simulink model "simulink_tri_motor_drone"  (R2020a)
settings: Solver=VariableStepAuto  StartTime=0.0  StopTime=50  RelTol=1e-3
values from neighbouring files (symbols this model uses):
  airDensity = 1.225    [tri_drone.m]
  areaWheelFront = wheelHeight*wheelWidth    (= 0.004)    [tri_drone.m]
  areaWing = 0.121    [tri_drone.m]
  cDFront = 0.9    [tri_drone.m]
  cDtable = [0.174 0.157 0.141 0.127 0.113 0.100 0.088 0.077 0.067 0.058 0.051 0.044 0.038 0.033 0.028 0.025 0.023 0.021 0.020 0.020 0.021 0.023 0.026 0.029 0.033 0.038 0.043 0.050 0.056 0.064 0.072 0.081 0.091 0.101 0.112 0.124 0.137 0.150 0.165 0.180 0.196 0.212 0.229 0.245 0.261 0.277 0.292 0.306 0.319 0.331 0.341]    [tri_drone.m]
  cLtable = [-1.07 -1.02 -0.97 -0.92 -0.87 -0.81 -0.76 -0.70 -0.65 -0.59 -0.54 -0.48 -0.43 -0.37 -0.31 -0.25 -0.19 -0.13 -0.07 -0.01 0.05 0.11 0.17 0.23 0.29 0.35 0.40 0.46 0.52 0.57 0.63 0.68 0.74 0.79 0.85 0.90 0.95 1.00 1.05 1.10 1.15 1.20 1.25 1.29 1.32 1.36 1.38 1.41 1.43 1.44 1.45]    [tri_drone.m]
  heightRef = 1.0    (= 1)    [tri_drone.m]
  hoverRot = w(11)    [tri_drone.m]
  hoverVel = trustPerPropeller / Ktrust /pi * 180.0    [tri_drone.m]
  hoverVoltagefine = 0.35*11.9    (= 4.165)    [tri_drone.m]
  KDheightcoarse = 15.0    (= 15)    [tri_drone.m]
  KDheightfine = 0    [tri_drone.m]
  KDrag = 8 * (ampMax * Km / (rpmMax / 60 * 2 * pi))    (= 0.000150440801971)    [tri_drone.m]
  KIheightcoarse = 5.0    (= 5)    [tri_drone.m]
  KIheightfine = 0    [tri_drone.m]
  Km = 60/(Kv * 2 * pi)    (= 0.00415186808066)    [tri_drone.m]
  KPheightcoarse = 0.1    [tri_drone.m]
  KPheightfine = 0    [tri_drone.m]
  Ktrust = (trustMax * g)/(rpmMax / 60 * 2 * pi)    (= 0.00223215912077)    [tri_drone.m]
  mBodyTotal = 0.422 + mBattery    (= 0.797)    [tri_drone.m]
  motorMass = 0.022    [tri_drone.m]
  N = 1000000    [tri_drone.m]
  pitch_lower_limit = theta(1)    [tri_drone.m]
  pitch_upper_limit = theta(end)    [tri_drone.m]
  propellerMass = 0.012    [tri_drone.m]
  Ra = RaVolt/ampMax    (= 0.133333333333)    [tri_drone.m]
  rInner = armRadius    (= 0.27)    [tri_drone.m]
  rOuter = armRadius + wLength    (= 0.91)    [tri_drone.m]
  theta = [-10 -9.5 -9.0 -8.5 -8.0 -7.5 -7.0 -6.5 -6.0 -5.5 -5.0 -4.5 -4.0 -3.5 -3.0 -2.5 -2.0 -1.5 -1.0 -0.5 0 0.5 1.0 1.5 2.0 2.5 3.0 3.5 4.0 4.5 5.0 5.5 6.0 6.5 7.0 7.5 8.0 8.5 9.0 9.5 10.0 10.5 11.0 11.5 12.0 12.5 13.0 13.5 14.0 14.5 15.0]    [tri_drone.m]
  Ts = 0.002    [tri_drone.m]
  Ts2 = 0.03    [tri_drone.m]
  wHeight = 0.025    [tri_drone.m]
  wingDensity = 50    [tri_drone.m]
  wLength = 0.64    [tri_drone.m]
  wWidth = 0.20    (= 0.2)    [tri_drone.m]
undefined symbols (not defined in the file or in its folder): X, Y, Z
libraries: sm_lib x53, nesl_utility x45
(part 3 of 3)

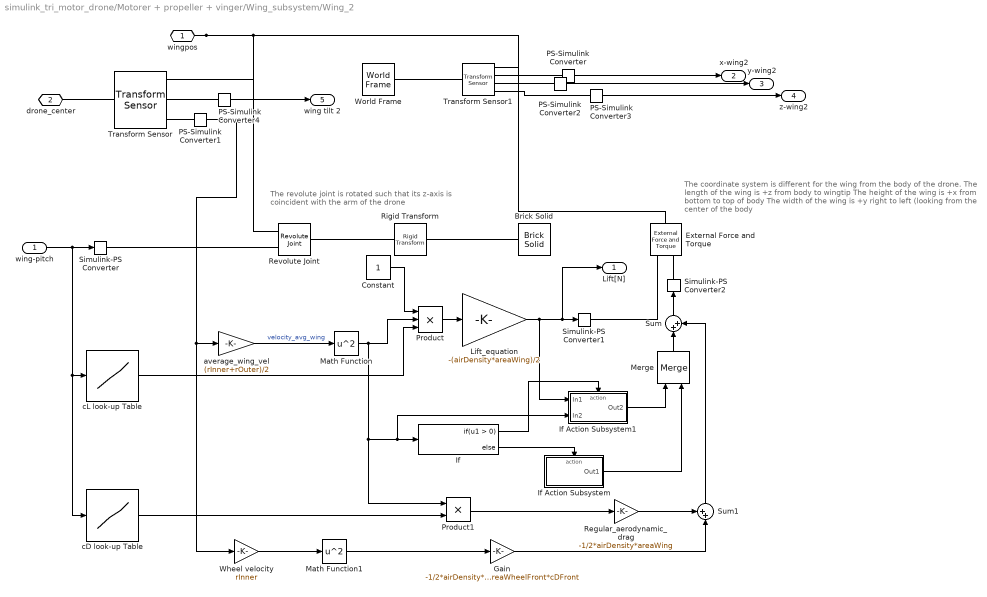
== system simulink_tri_motor_drone/Motorer + propeller + vinger/Wing_subsystem/Wing_2 ==
  note: The revolute joint is rotated such that its z-axis is
      | coincident with the arm of the drone
  note: The coordinate system is different for the wing from the body of the drone.
      | The length of the wing is +z from body to wingtip
      | The height of the wing is +x from bottom to top of body
      | The width of the wing is +y right to left (looking from the center of the body
  wing-pitch : Inport
  Brick Solid : sm_lib/Body Elements/Brick Solid  GraphicAmbientColor=[0.15 0.15 0.15 1.0]  BasedOnType=Mass  BrickDimensions=[wWidth wLength wHeight]  BrickDimensionUnits=m  CenterOfMass=[0 0 0]  CenterOfMassUnits=m  GraphicDiffuseColor=[1.0 0.0 0.2]  Density=wingDensity  DensityUnits=kg/m^3  DoExposeReferenceFrame=on  GraphicEmissiveColor=[0.0 0.0 0.0 1.0]  ExportEntireGeometry=off  SerializedFrames=<Frames/>  MarkerShape=Sphere  MarkerSize=10  GraphicType=FromGeometry  InertiaType=CalculateFromGeometry  Mass=areaWing*wHeight*wingDensity  MassUnits=kg  MomentsOfInertia=[1 1 1]  MomentsOfInertiaUnits=kg*m^2  GraphicOpacity=1.0  ProductsOfInertia=[0 0 0]  ProductsOfInertiaUnits=kg*m^2  GraphicShininess=75  GraphicSpecularColor=[0.5 0.5 0.5 1.0]  GraphicVisPropType=SimpleVisualProperties
  Constant : Constant
  External Force and Torque : sm_lib/Forces and Torques/External Force and Torque  ForceResolutionFrame=AttachedFrame  EnableForceX=on  EnableForceY=on  EnableForceZ=off  EnableForce=off  TorqueResolutionFrame=AttachedFrame  EnableTorqueX=off  EnableTorqueY=off  EnableTorqueZ=off  EnableTorque=off
  Gain : Gain  Gain=-1/2*airDensity*areaWheelFront*cDFront
  If : If
  If Action Subsystem : Subsystem  TreatAsAtomicUnit=on
  If Action Subsystem1 : Subsystem  TreatAsAtomicUnit=on
  Lift_equation : Gain  Gain=-(airDensity*areaWing)/2
  Math Function : Math  Operator=square  SaturateOnIntegerOverflow=on
  Math Function1 : Math  Operator=square  SaturateOnIntegerOverflow=on
  Merge : Merge
  PS-Simulink Converter{,1..4} (5 alike) : nesl_utility/PS-Simulink Converter  PhysicalDomain=network_engine_domain  SubClassName=ps_output  LeftPortType=input  RightPortType=output  PseudoPeriodic=off  Frequencies=[]  Unit=inherit  AffineConversion=off
  Product : Product  Inputs=3
  Product1 : Product
  Regular_aerodynamic_drag : Gain  Gain=-1/2*airDensity*areaWing
  Revolute Joint : sm_lib/Joints/Revolute Joint  JointMode=Normal  SenseConstraintForce=off  SenseConstraintForceX=off  SenseConstraintForceY=off  SenseConstraintForceZ=off  SenseConstraintTorque=off  SenseConstraintTorqueX=off  SenseConstraintTorqueY=off  SenseConstraintTorqueZ=off  SenseTotalForce=off  SenseTotalForceX=off  SenseTotalForceY=off  SenseTotalForceZ=off  SenseTotalTorque=off  SenseTotalTorqueX=off  SenseTotalTorqueY=off  SenseTotalTorqueZ=off  CompositeWrenchDir=FollowerOnBase  CompositeWrenchFrame=BaseFrame  EquilibriumPosition=0  EquilibriumPositionUnits=deg  SpringStiffness=0  SpringStiffnessUnits=N*m/deg  DampingCoefficient=0  DampingCoefficientUnits=N*m/(deg/s)  TorqueActuationMode=ComputedTorque  MotionActuationMode=InputMotion  SensePosition=off  SenseVelocity=off  SenseAcceleration=off  SenseTorqueForce=off  SenseLowerLimitTorqueForce=off  SenseUpperLimitTorqueForce=off  LowerLimitSpecify=off  LowerLimitBound=-90  LowerLimitBoundUnits=deg  LowerLimitStiffness=1e4  LowerLimitStiffnessUnits=N*m/deg  LowerLimitDamping=10  LowerLimitDampingUnits=N*m/(deg/s)  LowerLimitTransitionRegionWidth=0.1  LowerLimitTransitionRegionWidthUnits=deg  UpperLimitSpecify=off  UpperLimitBound=90  UpperLimitBoundUnits=deg  UpperLimitStiffness=1e4  UpperLimitStiffnessUnits=N*m/deg  UpperLimitDamping=10  UpperLimitDampingUnits=N*m/(deg/s)  UpperLimitTransitionRegionWidth=0.1  UpperLimitTransitionRegionWidthUnits=deg  PositionTargetSpecify=off  PositionTargetPriority=High  PositionTargetValue=0  PositionTargetValueUnits=deg  VelocityTargetSpecify=off  VelocityTargetPriority=High  VelocityTargetValue=0  VelocityTargetValueUnits=deg/s
  Rigid Transform : sm_lib/Frames and Transforms/Rigid Transform  TranslationMethod=Cartesian  TranslationStandardOffset=0  TranslationLengthUnit=m  TranslationStandardAxis=+Z  TranslationCartesianOffset=[0 0 wLength/2]  TranslationROffset=0  TranslationROffsetUnits=m  TranslationZOffset=0  TranslationZOffsetUnits=m  TranslationThetaOffset=0  TranslationThetaOffsetUnits=deg  RotationMethod=RotationSequence  RotationAngleUnits=deg  RotationStandardAxis=+Z  RotationAngle=0.0  RotationArbitraryAxis=[0 0 1]  FollAlignAxisA=+X  BaseAlignAxisA=+Y  FollAlignAxisB=+Y  BaseAlignAxisB=+Z  RotationSequenceAxes=FollowerAxes  RotationSequence=XZY  RotationSequenceAngles=[90 0 90]  RotationSequenceAnglesUnits=deg  RotationMatrix=[1 0 0; 0 1 0; 0 0 1]
  Simulink-PS Converter : nesl_utility/Simulink-PS Converter  PhysicalDomain=network_engine_domain  SubClassName=ps_input  LeftPortType=input  RightPortType=output  PseudoPeriodic=off  Frequencies=[]  NoiseDistribution=none  NoiseParameters=[]  Unit=deg  AffineConversion=off  FilteringAndDerivatives=filter  SimscapeFilterOrder=2  InputFilterTimeConstant=0.001  UdotUserProvided=0
  Simulink-PS Converter1 : nesl_utility/Simulink-PS Converter  PhysicalDomain=network_engine_domain  SubClassName=ps_input  LeftPortType=input  RightPortType=output  PseudoPeriodic=off  Frequencies=[]  NoiseDistribution=none  NoiseParameters=[]  Unit=1  AffineConversion=off  FilteringAndDerivatives=provide  SimscapeFilterOrder=1  InputFilterTimeConstant=0.001  UdotUserProvided=0
  Simulink-PS Converter2 : nesl_utility/Simulink-PS Converter  PhysicalDomain=network_engine_domain  SubClassName=ps_input  LeftPortType=input  RightPortType=output  PseudoPeriodic=off  Frequencies=[]  NoiseDistribution=none  NoiseParameters=[]  Unit=1  AffineConversion=off  FilteringAndDerivatives=provide  SimscapeFilterOrder=1  InputFilterTimeConstant=0.001  UdotUserProvided=0
  Sum : Sum  Inputs=|++
  Sum1 : Sum  Inputs=++|
  Transform Sensor : sm_lib/Frames and Transforms/Transform Sensor  MeasurementFrame=World  SenseAngle=on  SenseAxis=off  SenseAngle1=off  SenseAngle2=off  SenseAngle3=off  SenseQ=off  SenseR=off  SenseOmegaX=off  SenseOmegaY=off  SenseOmegaZ=on  SenseOmega1=off  SenseOmega2=off  SenseOmega3=off  SenseQDot=off  SenseRDot=off  SenseAlphaX=off  SenseAlphaY=off  SenseAlphaZ=off  SenseAlpha1=off  SenseAlpha2=off  SenseAlpha3=off  SenseQDDot=off  SenseRDDot=off  SenseX=off  SenseY=off  SenseZ=off  SenseRad=off  SenseAzim=off  SenseDist=off  SenseInc=off  SenseXDot=off  SenseYDot=off  SenseZDot=off  SenseRadDot=off  SenseAzimDot=off  SenseDistDot=off  SenseIncDot=off  SenseXDDot=off  SenseYDDot=off  SenseZDDot=off  SenseRadDDot=off  SenseAzimDDot=off  SenseDistDDot=off  SenseIncDDot=off
  Transform Sensor1 : sm_lib/Frames and Transforms/Transform Sensor  MeasurementFrame=World  SenseAngle=off  SenseAxis=off  SenseAngle1=off  SenseAngle2=off  SenseAngle3=off  SenseQ=off  SenseR=off  SenseOmegaX=off  SenseOmegaY=off  SenseOmegaZ=off  SenseOmega1=off  SenseOmega2=off  SenseOmega3=off  SenseQDot=off  SenseRDot=off  SenseAlphaX=off  SenseAlphaY=off  SenseAlphaZ=off  SenseAlpha1=off  SenseAlpha2=off  SenseAlpha3=off  SenseQDDot=off  SenseRDDot=off  SenseX=on  SenseY=on  SenseZ=on  SenseRad=off  SenseAzim=off  SenseDist=off  SenseInc=off  SenseXDot=off  SenseYDot=off  SenseZDot=off  SenseRadDot=off  SenseAzimDot=off  SenseDistDot=off  SenseIncDot=off  SenseXDDot=off  SenseYDDot=off  SenseZDDot=off  SenseRadDDot=off  SenseAzimDDot=off  SenseDistDDot=off  SenseIncDDot=off
  Wheel velocity : Gain  Gain=rInner
  World Frame : sm_lib/Frames and Transforms/World Frame
  average_wing_vel : Gain  Gain=(rInner+rOuter)/2
  cD look-up Table : Lookup_n-D  NumberOfTableDimensions=1  BreakpointsForDimension1=theta  Table=cDtable  InternalRulePriority=Speed  RndMeth=Simplest  InputSameDT=on
  cL look-up Table : Lookup_n-D  NumberOfTableDimensions=1  BreakpointsForDimension1=theta  Table=cLtable  InternalRulePriority=Speed  RndMeth=Simplest  InputSameDT=on
  wingpos : PMIOPort  Side=Left
  drone_center : PMIOPort  Port=2  Side=Left
  Lift[N] : Outport
  x-wing2 : Outport  Port=2
  y-wing2 : Outport  Port=3
  z-wing2 : Outport  Port=4
  wing tilt 2 : Outport  Port=5
  wires:
  wing-pitch/1 -> cD look-up Table/1, cL look-up Table/1, Simulink-PS Converter/1
  average_wing_vel/1 -> Math Function/1  "velocity_avg_wing"
  Product/1 -> Lift_equation/1
  PS-Simulink Converter/1 -> x-wing2/1
  PS-Simulink Converter2/1 -> y-wing2/1
  PS-Simulink Converter3/1 -> z-wing2/1
  cL look-up Table/1 -> Product/3
  Math Function/1 -> Product1/1, If Action Subsystem1/2(In2), If/1, Product/2
  If/1 -> If Action Subsystem1/Action
  If/2 -> If Action Subsystem/Action
  If Action Subsystem/1(Out1) -> Merge/2
  If Action Subsystem1/1(Out2) -> Merge/1
  Lift_equation/1 -> If Action Subsystem1/1(In1), Lift[N]/1, Simulink-PS Converter1/1
  Sum/1 -> Simulink-PS Converter2/1
  Merge/1 -> Sum/1
  PS-Simulink Converter4/1 -> wing tilt 2/1
  cD look-up Table/1 -> Product1/2
  Product1/1 -> Regular_aerodynamic_drag/1
  Constant/1 -> Product/1
  Gain/1 -> Sum1/2
  Wheel velocity/1 -> Math Function1/1
  PS-Simulink Converter1/1 -> Wheel velocity/1, average_wing_vel/1
  Math Function1/1 -> Gain/1
  Regular_aerodynamic_drag/1 -> Sum1/1
  Sum1/1 -> Sum/2
  connections:
  wingpos/RConn1 -- External Force and Torque/RConn1 -- Transform Sensor1/RConn1 -- Revolute Joint/LConn1 -- Transform Sensor/RConn1
  Revolute Joint/LConn2 -- Simulink-PS Converter/RConn1
  Rigid Transform/RConn1 -- Brick Solid/RConn1
  drone_center/RConn1 -- Transform Sensor/LConn1
  External Force and Torque/LConn1 -- Simulink-PS Converter1/RConn1
  World Frame/RConn1 -- Transform Sensor1/LConn1
  PS-Simulink Converter/LConn1 -- Transform Sensor1/RConn2
  Transform Sensor1/RConn3 -- PS-Simulink Converter2/LConn1
  Transform Sensor1/RConn4 -- PS-Simulink Converter3/LConn1
  Rigid Transform/LConn1 -- Revolute Joint/RConn1
  Simulink-PS Converter2/RConn1 -- External Force and Torque/LConn2
  Transform Sensor/RConn3 -- PS-Simulink Converter1/LConn1
  Transform Sensor/RConn2 -- PS-Simulink Converter4/LConn1

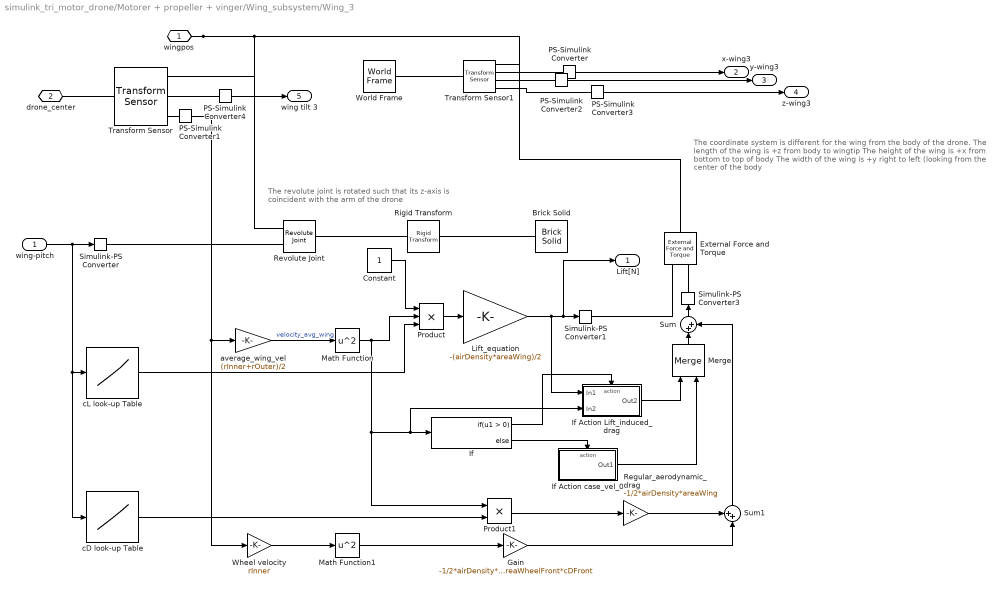
== system simulink_tri_motor_drone/Motorer + propeller + vinger/Wing_subsystem/Wing_3 ==
  note: The revolute joint is rotated such that its z-axis is
      | coincident with the arm of the drone
  note: The coordinate system is different for the wing from the body of the drone.
      | The length of the wing is +z from body to wingtip
      | The height of the wing is +x from bottom to top of body
      | The width of the wing is +y right to left (looking from the center of the body
  wing-pitch : Inport
  Brick Solid : sm_lib/Body Elements/Brick Solid  GraphicAmbientColor=[0.15 0.15 0.15 1.0]  BasedOnType=Mass  BrickDimensions=[wWidth wLength wHeight]  BrickDimensionUnits=m  CenterOfMass=[0 0 0]  CenterOfMassUnits=m  GraphicDiffuseColor=[1.0 0.8 0.0]  Density=wingDensity  DensityUnits=kg/m^3  DoExposeReferenceFrame=on  GraphicEmissiveColor=[0.0 0.0 0.0 1.0]  ExportEntireGeometry=off  SerializedFrames=<Frames/>  MarkerShape=Sphere  MarkerSize=10  GraphicType=FromGeometry  InertiaType=CalculateFromGeometry  Mass=areaWing*wHeight*wingDensity  MassUnits=kg  MomentsOfInertia=[1 1 1]  MomentsOfInertiaUnits=kg*m^2  GraphicOpacity=1.0  ProductsOfInertia=[0 0 0]  ProductsOfInertiaUnits=kg*m^2  GraphicShininess=75  GraphicSpecularColor=[0.5 0.5 0.5 1.0]  GraphicVisPropType=SimpleVisualProperties
  Constant : Constant
  External Force and Torque : sm_lib/Forces and Torques/External Force and Torque  ForceResolutionFrame=AttachedFrame  EnableForceX=on  EnableForceY=on  EnableForceZ=off  EnableForce=off  TorqueResolutionFrame=AttachedFrame  EnableTorqueX=off  EnableTorqueY=off  EnableTorqueZ=off  EnableTorque=off
  Gain : Gain  Gain=-1/2*airDensity*areaWheelFront*cDFront
  If : If
  If Action Lift_induced_drag : Subsystem  TreatAsAtomicUnit=on
  If Action case_vel_0 : Subsystem  TreatAsAtomicUnit=on
  Lift_equation : Gain  Gain=-(airDensity*areaWing)/2
  Math Function : Math  Operator=square  SaturateOnIntegerOverflow=on
  Math Function1 : Math  Operator=square  SaturateOnIntegerOverflow=on
  Merge : Merge  InitialOutput=0
  PS-Simulink Converter{,1..4} (5 alike) : nesl_utility/PS-Simulink Converter  PhysicalDomain=network_engine_domain  SubClassName=ps_output  LeftPortType=input  RightPortType=output  PseudoPeriodic=off  Frequencies=[]  Unit=inherit  AffineConversion=off
  Product : Product  Inputs=3
  Product1 : Product
  Regular_aerodynamic_drag : Gain  Gain=-1/2*airDensity*areaWing
  Revolute Joint : sm_lib/Joints/Revolute Joint  JointMode=Normal  SenseConstraintForce=off  SenseConstraintForceX=off  SenseConstraintForceY=off  SenseConstraintForceZ=off  SenseConstraintTorque=off  SenseConstraintTorqueX=off  SenseConstraintTorqueY=off  SenseConstraintTorqueZ=off  SenseTotalForce=off  SenseTotalForceX=off  SenseTotalForceY=off  SenseTotalForceZ=off  SenseTotalTorque=off  SenseTotalTorqueX=off  SenseTotalTorqueY=off  SenseTotalTorqueZ=off  CompositeWrenchDir=FollowerOnBase  CompositeWrenchFrame=BaseFrame  EquilibriumPosition=0  EquilibriumPositionUnits=deg  SpringStiffness=0  SpringStiffnessUnits=N*m/deg  DampingCoefficient=0  DampingCoefficientUnits=N*m/(deg/s)  TorqueActuationMode=ComputedTorque  MotionActuationMode=InputMotion  SensePosition=off  SenseVelocity=off  SenseAcceleration=off  SenseTorqueForce=off  SenseLowerLimitTorqueForce=off  SenseUpperLimitTorqueForce=off  LowerLimitSpecify=off  LowerLimitBound=-90  LowerLimitBoundUnits=deg  LowerLimitStiffness=1e4  LowerLimitStiffnessUnits=N*m/deg  LowerLimitDamping=10  LowerLimitDampingUnits=N*m/(deg/s)  LowerLimitTransitionRegionWidth=0.1  LowerLimitTransitionRegionWidthUnits=deg  UpperLimitSpecify=off  UpperLimitBound=90  UpperLimitBoundUnits=deg  UpperLimitStiffness=1e4  UpperLimitStiffnessUnits=N*m/deg  UpperLimitDamping=10  UpperLimitDampingUnits=N*m/(deg/s)  UpperLimitTransitionRegionWidth=0.1  UpperLimitTransitionRegionWidthUnits=deg  PositionTargetSpecify=off  PositionTargetPriority=High  PositionTargetValue=0  PositionTargetValueUnits=deg  VelocityTargetSpecify=off  VelocityTargetPriority=High  VelocityTargetValue=0  VelocityTargetValueUnits=deg/s
  Rigid Transform : sm_lib/Frames and Transforms/Rigid Transform  TranslationMethod=Cartesian  TranslationStandardOffset=0  TranslationLengthUnit=m  TranslationStandardAxis=+Z  TranslationCartesianOffset=[0 0 wLength/2]  TranslationROffset=0  TranslationROffsetUnits=m  TranslationZOffset=0  TranslationZOffsetUnits=m  TranslationThetaOffset=0  TranslationThetaOffsetUnits=deg  RotationMethod=RotationSequence  RotationAngleUnits=deg  RotationStandardAxis=+Z  RotationAngle=0.0  RotationArbitraryAxis=[0 0 1]  FollAlignAxisA=+X  BaseAlignAxisA=+Y  FollAlignAxisB=+Y  BaseAlignAxisB=+Z  RotationSequenceAxes=FollowerAxes  RotationSequence=XZY  RotationSequenceAngles=[90 0 90]  RotationSequenceAnglesUnits=deg  RotationMatrix=[1 0 0; 0 1 0; 0 0 1]
  Simulink-PS Converter : nesl_utility/Simulink-PS Converter  PhysicalDomain=network_engine_domain  SubClassName=ps_input  LeftPortType=input  RightPortType=output  PseudoPeriodic=off  Frequencies=[]  NoiseDistribution=none  NoiseParameters=[]  Unit=deg  AffineConversion=off  FilteringAndDerivatives=filter  SimscapeFilterOrder=2  InputFilterTimeConstant=0.001  UdotUserProvided=0
  Simulink-PS Converter1 : nesl_utility/Simulink-PS Converter  PhysicalDomain=network_engine_domain  SubClassName=ps_input  LeftPortType=input  RightPortType=output  PseudoPeriodic=off  Frequencies=[]  NoiseDistribution=none  NoiseParameters=[]  Unit=1  AffineConversion=off  FilteringAndDerivatives=provide  SimscapeFilterOrder=1  InputFilterTimeConstant=0.001  UdotUserProvided=0
  Simulink-PS Converter3 : nesl_utility/Simulink-PS Converter  PhysicalDomain=network_engine_domain  SubClassName=ps_input  LeftPortType=input  RightPortType=output  PseudoPeriodic=off  Frequencies=[]  NoiseDistribution=none  NoiseParameters=[]  Unit=1  AffineConversion=off  FilteringAndDerivatives=provide  SimscapeFilterOrder=1  InputFilterTimeConstant=0.001  UdotUserProvided=0
  Sum : Sum  Inputs=|++
  Sum1 : Sum  Inputs=++|
  Transform Sensor : sm_lib/Frames and Transforms/Transform Sensor  MeasurementFrame=Base  SenseAngle=on  SenseAxis=off  SenseAngle1=off  SenseAngle2=off  SenseAngle3=off  SenseQ=off  SenseR=off  SenseOmegaX=off  SenseOmegaY=off  SenseOmegaZ=on  SenseOmega1=off  SenseOmega2=off  SenseOmega3=off  SenseQDot=off  SenseRDot=off  SenseAlphaX=off  SenseAlphaY=off  SenseAlphaZ=off  SenseAlpha1=off  SenseAlpha2=off  SenseAlpha3=off  SenseQDDot=off  SenseRDDot=off  SenseX=off  SenseY=off  SenseZ=off  SenseRad=off  SenseAzim=off  SenseDist=off  SenseInc=off  SenseXDot=off  SenseYDot=off  SenseZDot=off  SenseRadDot=off  SenseAzimDot=off  SenseDistDot=off  SenseIncDot=off  SenseXDDot=off  SenseYDDot=off  SenseZDDot=off  SenseRadDDot=off  SenseAzimDDot=off  SenseDistDDot=off  SenseIncDDot=off
  Transform Sensor1 : sm_lib/Frames and Transforms/Transform Sensor  MeasurementFrame=World  SenseAngle=off  SenseAxis=off  SenseAngle1=off  SenseAngle2=off  SenseAngle3=off  SenseQ=off  SenseR=off  SenseOmegaX=off  SenseOmegaY=off  SenseOmegaZ=off  SenseOmega1=off  SenseOmega2=off  SenseOmega3=off  SenseQDot=off  SenseRDot=off  SenseAlphaX=off  SenseAlphaY=off  SenseAlphaZ=off  SenseAlpha1=off  SenseAlpha2=off  SenseAlpha3=off  SenseQDDot=off  SenseRDDot=off  SenseX=on  SenseY=on  SenseZ=on  SenseRad=off  SenseAzim=off  SenseDist=off  SenseInc=off  SenseXDot=off  SenseYDot=off  SenseZDot=off  SenseRadDot=off  SenseAzimDot=off  SenseDistDot=off  SenseIncDot=off  SenseXDDot=off  SenseYDDot=off  SenseZDDot=off  SenseRadDDot=off  SenseAzimDDot=off  SenseDistDDot=off  SenseIncDDot=off
  Wheel velocity : Gain  Gain=rInner
  World Frame : sm_lib/Frames and Transforms/World Frame
  average_wing_vel : Gain  Gain=(rInner+rOuter)/2
  cD look-up Table : Lookup_n-D  NumberOfTableDimensions=1  BreakpointsForDimension1=theta  Table=cDtable  InternalRulePriority=Speed  RndMeth=Simplest  InputSameDT=on
  cL look-up Table : Lookup_n-D  NumberOfTableDimensions=1  BreakpointsForDimension1=theta  Table=cLtable  InternalRulePriority=Speed  RndMeth=Simplest  InputSameDT=on
  wingpos : PMIOPort  Side=Left
  drone_center : PMIOPort  Port=2  Side=Left
  Lift[N] : Outport
  x-wing3 : Outport  Port=2
  y-wing3 : Outport  Port=3
  z-wing3 : Outport  Port=4
  wing tilt 3 : Outport  Port=5
  wires:
  wing-pitch/1 -> cD look-up Table/1, cL look-up Table/1, Simulink-PS Converter/1
  average_wing_vel/1 -> Math Function/1  "velocity_avg_wing"
  Product/1 -> Lift_equation/1
  PS-Simulink Converter/1 -> x-wing3/1
  PS-Simulink Converter2/1 -> y-wing3/1
  PS-Simulink Converter3/1 -> z-wing3/1
  cL look-up Table/1 -> Product/3
  If Action Lift_induced_drag/1(Out2) -> Merge/1
  Math Function/1 -> Product1/1, If Action Lift_induced_drag/2(In2), If/1, Product/2
  If Action case_vel_0/1(Out1) -> Merge/2
  If/2 -> If Action case_vel_0/Action
  If/1 -> If Action Lift_induced_drag/Action
  Lift_equation/1 -> If Action Lift_induced_drag/1(In1), Lift[N]/1, Simulink-PS Converter1/1
  Sum/1 -> Simulink-PS Converter3/1
  Merge/1 -> Sum/1
  PS-Simulink Converter4/1 -> wing tilt 3/1
  Product1/1 -> Regular_aerodynamic_drag/1
  cD look-up Table/1 -> Product1/2
  Constant/1 -> Product/1
  Wheel velocity/1 -> Math Function1/1
  PS-Simulink Converter1/1 -> Wheel velocity/1, average_wing_vel/1
  Math Function1/1 -> Gain/1
  Regular_aerodynamic_drag/1 -> Sum1/1
  Gain/1 -> Sum1/2
  Sum1/1 -> Sum/2
  connections:
  wingpos/RConn1 -- External Force and Torque/RConn1 -- Transform Sensor1/RConn1 -- Revolute Joint/LConn1 -- Transform Sensor/RConn1
  drone_center/RConn1 -- Transform Sensor/LConn1
  External Force and Torque/LConn1 -- Simulink-PS Converter1/RConn1
  World Frame/RConn1 -- Transform Sensor1/LConn1
  PS-Simulink Converter/LConn1 -- Transform Sensor1/RConn2
  Transform Sensor1/RConn3 -- PS-Simulink Converter2/LConn1
  Transform Sensor1/RConn4 -- PS-Simulink Converter3/LConn1
  Brick Solid/RConn1 -- Rigid Transform/RConn1
  Revolute Joint/LConn2 -- Simulink-PS Converter/RConn1
  Revolute Joint/RConn1 -- Rigid Transform/LConn1
  Simulink-PS Converter3/RConn1 -- External Force and Torque/LConn2
  PS-Simulink Converter1/LConn1 -- Transform Sensor/RConn3
  PS-Simulink Converter4/LConn1 -- Transform Sensor/RConn2

== system simulink_tri_motor_drone/Motorer + propeller + vinger/Wing_subsystem/Wing_1/If Action Subsystem ==
  Action Port : ActionPort  ActionPortLabel=else
  Constant : Constant  Value=0
  Out1 : Outport
  wires:
  Constant/1 -> Out1/1

== system simulink_tri_motor_drone/Motorer + propeller + vinger/Wing_subsystem/Wing_1/If Action Subsystem1 ==
  In1 : Inport
  In2 : Inport  Port=2
  Action Port : ActionPort  ActionPortLabel=if(u1 > 0)
  Divide : Product  Inputs=*/
  Math Function1 : Math  Operator=square  SaturateOnIntegerOverflow=on
  lift_induced_drag : Gain  Gain=-1/(0.5*airDensity*pi*(wLength^2))
  Out2 : Outport
  wires:
  lift_induced_drag/1 -> Out2/1
  Divide/1 -> lift_induced_drag/1
  Math Function1/1 -> Divide/1
  In2/1 -> Divide/2
  In1/1 -> Math Function1/1

== system simulink_tri_motor_drone/Motorer + propeller + vinger/Wing_subsystem/Wing_2/If Action Subsystem ==
  Action Port : ActionPort  ActionPortLabel=else
  Constant : Constant  Value=0
  Out1 : Outport
  wires:
  Constant/1 -> Out1/1

== system simulink_tri_motor_drone/Motorer + propeller + vinger/Wing_subsystem/Wing_2/If Action Subsystem1 ==
  In1 : Inport
  In2 : Inport  Port=2
  Action Port : ActionPort  ActionPortLabel=if(u1 > 0)
  Divide : Product  Inputs=*/
  Math Function1 : Math  Operator=square  SaturateOnIntegerOverflow=on
  lift_induced_drag : Gain  Gain=-1/(0.5*airDensity*pi*(wLength^2))
  Out2 : Outport
  wires:
  lift_induced_drag/1 -> Out2/1
  Divide/1 -> lift_induced_drag/1
  Math Function1/1 -> Divide/1
  In2/1 -> Divide/2
  In1/1 -> Math Function1/1

== system simulink_tri_motor_drone/Motorer + propeller + vinger/Wing_subsystem/Wing_3/If Action Lift_induced_drag ==
  In1 : Inport
  In2 : Inport  Port=2
  Action Port : ActionPort  ActionPortLabel=if(u1 > 0)
  Divide : Product  Inputs=*/
  Math Function1 : Math  Operator=square  SaturateOnIntegerOverflow=on
  lift_induced_drag : Gain  Gain=-1/(0.5*airDensity*pi*(wLength^2))
  Out2 : Outport
  wires:
  lift_induced_drag/1 -> Out2/1
  Divide/1 -> lift_induced_drag/1
  Math Function1/1 -> Divide/1
  In2/1 -> Divide/2
  In1/1 -> Math Function1/1

== system simulink_tri_motor_drone/Motorer + propeller + vinger/Wing_subsystem/Wing_3/If Action case_vel_0 ==
  Action Port : ActionPort  ActionPortLabel=else
  Constant : Constant  Value=0
  Out1 : Outport
  wires:
  Constant/1 -> Out1/1
